simulink model "A4a"  (R2018a)
settings: Solver=VariableStepAuto  StartTime=0.0  StopTime=50  RelTol=1e-3
settings Model: Creator=U500304  LastModifiedBy=U500304

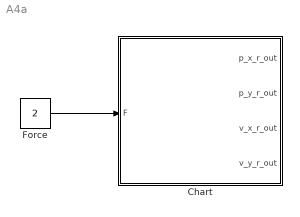
== system A4a ==
  Chart : Stateflow chart  TreatAsAtomicUnit=on
  Force : Constant  Value=2
  wires:
  Force/1 -> Chart/1(F)

== stateflow chart A4a/Chart ==
  state Robot
    en,du:
    % Robot
    p_x_r_dot = v_x_r;
    p_y_r_dot = 0;
    v_x_r_dot = F / m_r;
    v_y_r_dot = 0;
    % Ball
    p_x_b_dot = 0;
    p_y_b_dot = 0;
    v_x_b_dot = 0;
    v_y_b_dot = 0;
  state With_Ball
    en:
    p_x_r_out = p_x_r;
    p_y_r_out = p_y_r;
    v_x_r_out = v_x_r;
    v_y_r_out = v_y_r;
  (default) -> Robot : {
      | % Robot Position
      | p_x_r = 0;
      | p_y_r = 10;
      |
      | % Robot Velocity
      | v_x_r = 0;
      | v_y_r = 0;
      |
      | % Ball Position
      | p_x_b = 10;
      | p_y_b = 10;
      |
      | % Ball Velocity
      | v_x_b = 0;
      | v_y_b = 0;
      |
      | }
  Robot -> With_Ball : [p_x_r > 10]{v_x_r = v_x_r / 3}
  data: g constant double =9.81; m_r constant double =0.5; F input; p_x_r local; p_x_r_dot local; p_y_r local; v_x_r_dot local; v_y_r local; v_x_r local; p_x_b local; p_y_b local; v_x_b local; v_y_b local; m_b constant double =1; p_x_b_dot local; p_y_b_dot local; p_y_r_dot local; v_x_b_dot local; v_y_b_dot local; v_y_r_dot local; p_x_r_out output; p_y_r_out output; v_x_r_out output; v_y_r_out output
